simulink model "example2"  (R2019b)
settings: Solver=VariableStepAuto  StartTime=0.0  StopTime=10.0  RelTol=1e-3
settings Model: Creator=davis  LastModifiedBy=davis

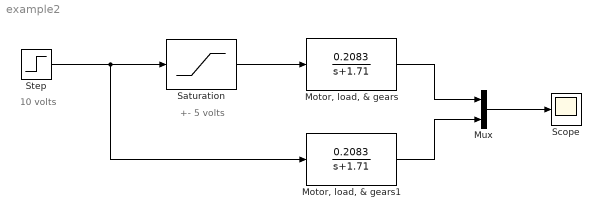
== system example2 ==
  note: +- 5 volts
  note: 10 volts
  "Motor, load, & gears" : TransferFcn  Numerator=[0.2083]  Denominator=[1 1.71]
  "Motor, load, & gears1" : TransferFcn  Numerator=[0.2083]  Denominator=[1 1.71]
  Mux : Mux  Inputs=2
  Saturation : Saturate  UpperLimit=5  LowerLimit=-5
  Scope : Scope
  Step : Step  Time=0  After=10  SampleTime=0
  wires:
  Step/1 -> "Motor, load, & gears1"/1, Saturation/1
  Saturation/1 -> "Motor, load, & gears"/1
  "Motor, load, & gears"/1 -> Mux/1
  "Motor, load, & gears1"/1 -> Mux/2
  Mux/1 -> Scope/1
